simulink model "PortMapTest"  (R2019b)
settings: Solver=FixedStepDiscrete  StartTime=0.0  StopTime=10.0  FixedStep=0.02  RelTol=1e-3
libraries: hdlsllib x4
settings Model: Creator=Yinglongli  LastModifiedBy=Yinglongli
settings OptimizationCC: OptimizeBlockIOStorage=off  BufferReuse=off  GlobalBufferReuse=off  ExpressionFolding=off  LocalBlockOutputs=off  OptimizeDataStoreBuffers=off  BusAssignmentInplaceUpdate=off
settings DebuggingCC: SFUnexpectedBacktrackingDiag=warning  SFNoUnconditionalDefaultTransitionDiag=warning
settings RTWCC: GenerateReport=on  BuildConfiguration=Debug  LaunchReport=on
settings CodeAppCC: ForceParamTrailComments=on  MATLABSourceComments=on  EnableCustomComments=on
settings GRTTargetCC: CombineSignalStateStructs=on  SupportVariableSizeSignals=on  MultiInstanceErrorCode=Warning

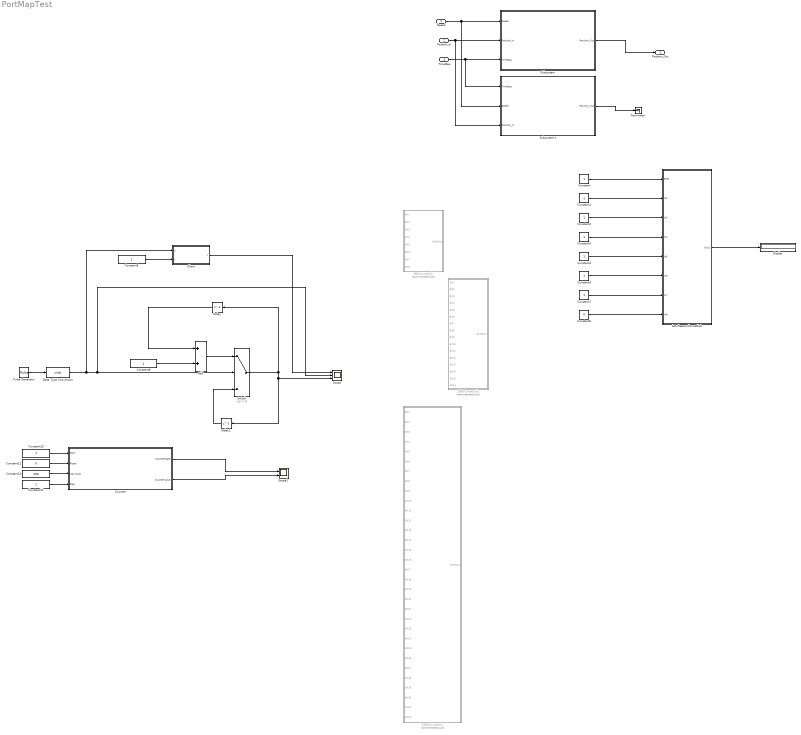
== system PortMapTest ==
  Speed : Inport
  Position_In : Inport  Port=2
  TimeGap : Inport  Port=3
  16BitConcatSub : Subsystem  Commented=on
  32BitConcatSub : Subsystem  Commented=on
  8BitConcatSub : Subsystem  Commented=on
  ActvReasonConcatSub : Subsystem  mask{numInputs=8}
      mask prompts: numInputs "Number of Inputs"
      mask TypeOptions numInputs: Bit Concat/numInputs
      mask Callback numInputs: parentInHandle = find_system(gcb,'FindAll','on','SearchDepth','1','BlockType','Inport');
      mask Display: disp('Bit Concatenation\n')
  Add : Sum
  Chart : Stateflow chart  BlockKeywords=__PRM__SERIALIZED__DATA__:Stateflow Chart,Stateflow Diagram  TreatAsAtomicUnit=on
  Constant{,1..5,7} (7 alike) : Constant  OutDataTypeStr=boolean
  Constant10 : Constant  Value=200  OutDataTypeStr=uint32
  Constant11 : Constant  OutDataTypeStr=uint8
  Constant12 : Constant  Value=0  OutDataTypeStr=uint8
  Constant13 : Constant  OutDataTypeStr=uint8
  Constant6 : Constant  Value=0  OutDataTypeStr=boolean
  Constant8 : Constant
  Constant9 : Constant  OutDataTypeStr=uint32
  Counter : Subsystem
  Data Type Conversion : DataTypeConversion  OutDataTypeStr=uint8
  Delay : Delay  DelayLength=1
  Delay1 : Delay  DelayLength=1
  Display : Display
      settings: Format=decimal (Stored Integer)
  Pulse Generator : DiscretePulseGenerator  PulseType=Time based  Period=0.04  PulseWidth=50
  Scope : Scope  NumInputPorts=3
  Scope1 : Scope  NumInputPorts=2
  Subsystem : Subsystem
  Subsystem1 : Subsystem
  Switch : Switch  Criteria=u2 > Threshold
  Terminator : Terminator
  Position_Out : Outport
  wires:
  Speed/1 -> Subsystem/1(Speed), Subsystem1/2(Speed)
  Position_In/1 -> Subsystem/2(Position_In), Subsystem1/3(Position_In)
  TimeGap/1 -> Subsystem/3(TimeGap), Subsystem1/1(TimeGap)
  Subsystem/1(Position_Out) -> Position_Out/1
  Subsystem1/1(Position_Out) -> Terminator/1
  Constant/1 -> ActvReasonConcatSub/1(Bit8)
  Constant1/1 -> ActvReasonConcatSub/2(In2)
  Constant2/1 -> ActvReasonConcatSub/3(In3)
  Constant3/1 -> ActvReasonConcatSub/4(In4)
  Constant4/1 -> ActvReasonConcatSub/5(In5)
  Constant5/1 -> ActvReasonConcatSub/6(In6)
  Constant7/1 -> ActvReasonConcatSub/7(In7)
  Constant6/1 -> ActvReasonConcatSub/8(In8)
  ActvReasonConcatSub/1(Out1) -> Display/1
  Constant8/1 -> Add/2
  Delay/1 -> Add/1
  Add/1 -> Switch/1
  Switch/1 -> Scope/3, Delay1/1, Delay/1
  Delay1/1 -> Switch/3
  Chart/1(y) -> Scope/1
  Pulse Generator/1 -> Data Type Conversion/1
  Constant9/1 -> Chart/2(t)
  Data Type Conversion/1 -> Chart/1(u), Scope/2, Switch/2
  Constant10/1 -> Counter/3(MaxValue)
  Constant11/1 -> Counter/4(Step)
  Constant12/1 -> Counter/2(Reset)
  Constant13/1 -> Counter/1(Start)
  Counter/1(CounterState) -> Scope1/1
  Counter/2(CounterValue) -> Scope1/2

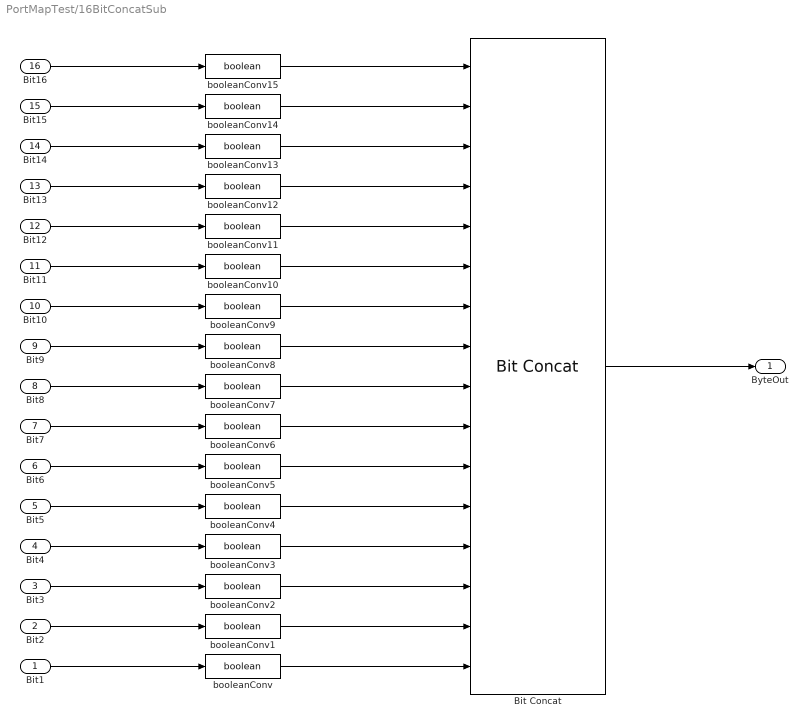
== system PortMapTest/16BitConcatSub ==
  Bit1 : Inport
  Bit2 : Inport  Port=2
  Bit3 : Inport  Port=3
  Bit4 : Inport  Port=4
  Bit5 : Inport  Port=5
  Bit6 : Inport  Port=6
  Bit7 : Inport  Port=7
  Bit8 : Inport  Port=8
  Bit9 : Inport  Port=9
  Bit10 : Inport  Port=10
  Bit11 : Inport  Port=11
  Bit12 : Inport  Port=12
  Bit13 : Inport  Port=13
  Bit14 : Inport  Port=14
  Bit15 : Inport  Port=15
  Bit16 : Inport  Port=16
  Bit Concat : hdlsllib/Logic and Bit Operations/Bit Concat  numInputs=16
      settings: SourceProductName=Simulink
  booleanConv{,1..15} (16 alike) : DataTypeConversion  OutDataTypeStr=boolean
  ByteOut : Outport
  wires:
  Bit Concat/1 -> ByteOut/1
  Bit8/1 -> booleanConv7/1
  Bit7/1 -> booleanConv6/1
  Bit6/1 -> booleanConv5/1
  Bit5/1 -> booleanConv4/1
  Bit4/1 -> booleanConv3/1
  Bit3/1 -> booleanConv2/1
  Bit2/1 -> booleanConv1/1
  Bit1/1 -> booleanConv/1
  booleanConv7/1 -> Bit Concat/9
  booleanConv6/1 -> Bit Concat/10
  booleanConv5/1 -> Bit Concat/11
  booleanConv4/1 -> Bit Concat/12
  booleanConv3/1 -> Bit Concat/13
  booleanConv2/1 -> Bit Concat/14
  booleanConv1/1 -> Bit Concat/15
  booleanConv/1 -> Bit Concat/16
  booleanConv15/1 -> Bit Concat/1
  booleanConv14/1 -> Bit Concat/2
  booleanConv13/1 -> Bit Concat/3
  booleanConv12/1 -> Bit Concat/4
  booleanConv11/1 -> Bit Concat/5
  booleanConv10/1 -> Bit Concat/6
  booleanConv9/1 -> Bit Concat/7
  booleanConv8/1 -> Bit Concat/8
  Bit16/1 -> booleanConv15/1
  Bit15/1 -> booleanConv14/1
  Bit14/1 -> booleanConv13/1
  Bit13/1 -> booleanConv12/1
  Bit12/1 -> booleanConv11/1
  Bit10/1 -> booleanConv9/1
  Bit11/1 -> booleanConv10/1
  Bit9/1 -> booleanConv8/1

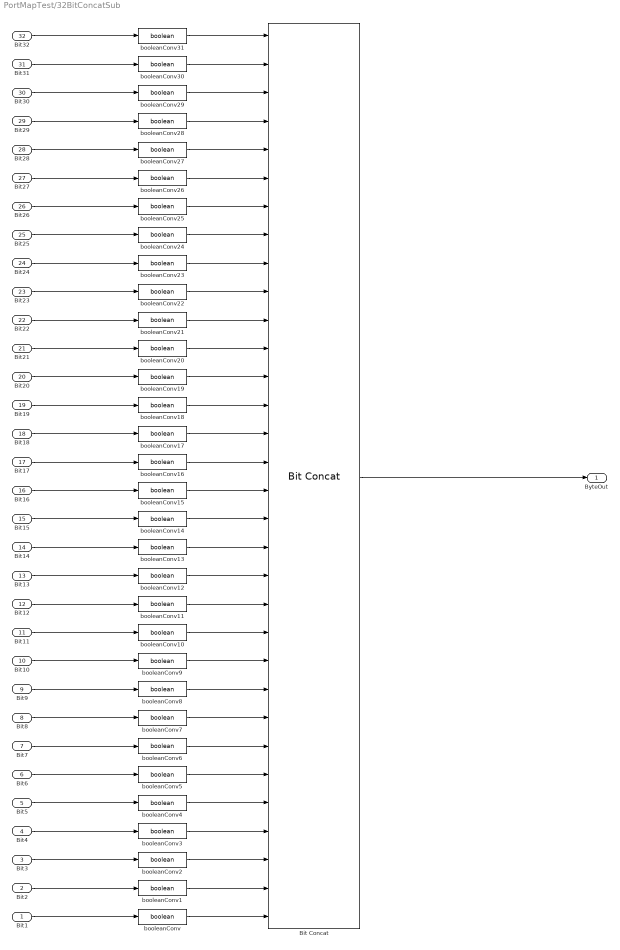
== system PortMapTest/32BitConcatSub ==
  Bit1 : Inport
  Bit2 : Inport  Port=2
  Bit3 : Inport  Port=3
  Bit4 : Inport  Port=4
  Bit5 : Inport  Port=5
  Bit6 : Inport  Port=6
  Bit7 : Inport  Port=7
  Bit8 : Inport  Port=8
  Bit9 : Inport  Port=9
  Bit10 : Inport  Port=10
  Bit11 : Inport  Port=11
  Bit12 : Inport  Port=12
  Bit13 : Inport  Port=13
  Bit14 : Inport  Port=14
  Bit15 : Inport  Port=15
  Bit16 : Inport  Port=16
  Bit17 : Inport  Port=17
  Bit18 : Inport  Port=18
  Bit19 : Inport  Port=19
  Bit20 : Inport  Port=20
  Bit21 : Inport  Port=21
  Bit22 : Inport  Port=22
  Bit23 : Inport  Port=23
  Bit24 : Inport  Port=24
  Bit25 : Inport  Port=25
  Bit26 : Inport  Port=26
  Bit27 : Inport  Port=27
  Bit28 : Inport  Port=28
  Bit29 : Inport  Port=29
  Bit30 : Inport  Port=30
  Bit31 : Inport  Port=31
  Bit32 : Inport  Port=32
  Bit Concat : hdlsllib/Logic and Bit Operations/Bit Concat  numInputs=32
      settings: SourceProductName=Simulink
  booleanConv{,1..31} (32 alike) : DataTypeConversion  OutDataTypeStr=boolean
  ByteOut : Outport
  wires:
  Bit Concat/1 -> ByteOut/1
  Bit8/1 -> booleanConv7/1
  Bit7/1 -> booleanConv6/1
  Bit6/1 -> booleanConv5/1
  Bit5/1 -> booleanConv4/1
  Bit4/1 -> booleanConv3/1
  Bit3/1 -> booleanConv2/1
  Bit2/1 -> booleanConv1/1
  Bit1/1 -> booleanConv/1
  Bit16/1 -> booleanConv15/1
  Bit15/1 -> booleanConv14/1
  Bit14/1 -> booleanConv13/1
  Bit13/1 -> booleanConv12/1
  Bit12/1 -> booleanConv11/1
  Bit10/1 -> booleanConv9/1
  Bit11/1 -> booleanConv10/1
  Bit9/1 -> booleanConv8/1
  booleanConv/1 -> Bit Concat/32
  booleanConv1/1 -> Bit Concat/31
  booleanConv2/1 -> Bit Concat/30
  booleanConv3/1 -> Bit Concat/29
  booleanConv4/1 -> Bit Concat/28
  booleanConv5/1 -> Bit Concat/27
  booleanConv6/1 -> Bit Concat/26
  booleanConv7/1 -> Bit Concat/25
  booleanConv8/1 -> Bit Concat/24
  booleanConv9/1 -> Bit Concat/23
  booleanConv10/1 -> Bit Concat/22
  booleanConv11/1 -> Bit Concat/21
  booleanConv12/1 -> Bit Concat/20
  booleanConv13/1 -> Bit Concat/19
  booleanConv14/1 -> Bit Concat/18
  booleanConv15/1 -> Bit Concat/17
  booleanConv31/1 -> Bit Concat/1
  booleanConv30/1 -> Bit Concat/2
  booleanConv29/1 -> Bit Concat/3
  booleanConv28/1 -> Bit Concat/4
  booleanConv27/1 -> Bit Concat/5
  booleanConv26/1 -> Bit Concat/6
  booleanConv25/1 -> Bit Concat/7
  booleanConv24/1 -> Bit Concat/8
  booleanConv23/1 -> Bit Concat/9
  booleanConv22/1 -> Bit Concat/10
  booleanConv21/1 -> Bit Concat/11
  booleanConv20/1 -> Bit Concat/12
  booleanConv19/1 -> Bit Concat/13
  booleanConv18/1 -> Bit Concat/14
  booleanConv17/1 -> Bit Concat/15
  booleanConv16/1 -> Bit Concat/16
  Bit17/1 -> booleanConv16/1
  Bit18/1 -> booleanConv17/1
  Bit19/1 -> booleanConv18/1
  Bit20/1 -> booleanConv19/1
  Bit21/1 -> booleanConv20/1
  Bit22/1 -> booleanConv21/1
  Bit23/1 -> booleanConv22/1
  Bit24/1 -> booleanConv23/1
  Bit25/1 -> booleanConv24/1
  Bit26/1 -> booleanConv25/1
  Bit27/1 -> booleanConv26/1
  Bit28/1 -> booleanConv27/1
  Bit29/1 -> booleanConv28/1
  Bit30/1 -> booleanConv29/1
  Bit31/1 -> booleanConv30/1
  Bit32/1 -> booleanConv31/1

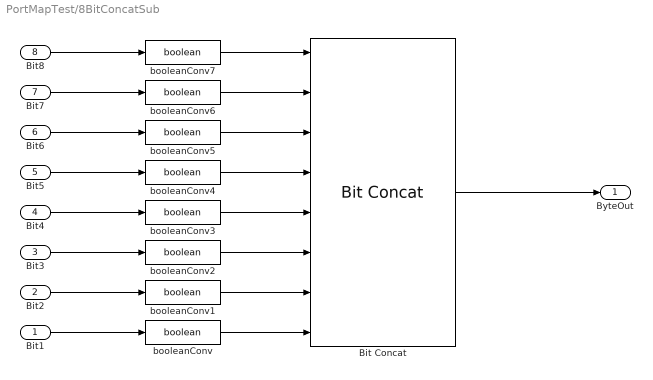
== system PortMapTest/8BitConcatSub ==
  Bit1 : Inport
  Bit2 : Inport  Port=2
  Bit3 : Inport  Port=3
  Bit4 : Inport  Port=4
  Bit5 : Inport  Port=5
  Bit6 : Inport  Port=6
  Bit7 : Inport  Port=7
  Bit8 : Inport  Port=8
  Bit Concat : hdlsllib/Logic and Bit Operations/Bit Concat  numInputs=8
      settings: SourceProductName=Simulink
  booleanConv{,1..7} (8 alike) : DataTypeConversion  OutDataTypeStr=boolean
  ByteOut : Outport
  wires:
  Bit Concat/1 -> ByteOut/1
  Bit8/1 -> booleanConv7/1
  Bit7/1 -> booleanConv6/1
  Bit6/1 -> booleanConv5/1
  Bit5/1 -> booleanConv4/1
  Bit4/1 -> booleanConv3/1
  Bit3/1 -> booleanConv2/1
  Bit2/1 -> booleanConv1/1
  Bit1/1 -> booleanConv/1
  booleanConv/1 -> Bit Concat/8
  booleanConv1/1 -> Bit Concat/7
  booleanConv2/1 -> Bit Concat/6
  booleanConv3/1 -> Bit Concat/5
  booleanConv4/1 -> Bit Concat/4
  booleanConv5/1 -> Bit Concat/3
  booleanConv6/1 -> Bit Concat/2
  booleanConv7/1 -> Bit Concat/1

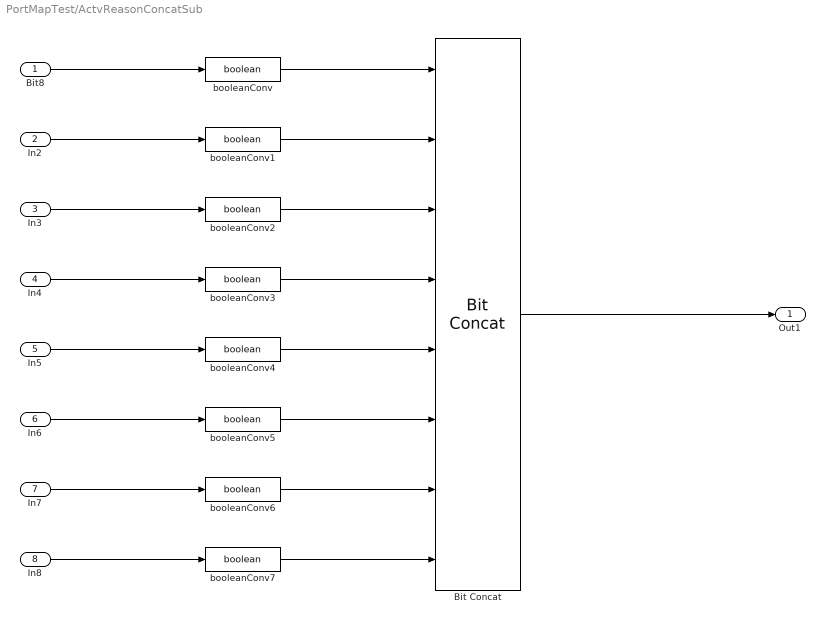
== system PortMapTest/ActvReasonConcatSub ==
  Bit8 : Inport
  In2 : Inport  Port=2
  In3 : Inport  Port=3
  In4 : Inport  Port=4
  In5 : Inport  Port=5
  In6 : Inport  Port=6
  In7 : Inport  Port=7
  In8 : Inport  Port=8
  Bit Concat : hdlsllib/Logic and Bit Operations/Bit Concat  numInputs=numInputs
      settings: SourceProductName=Simulink
  booleanConv{,1..7} (8 alike) : DataTypeConversion  OutDataTypeStr=boolean
  Out1 : Outport
  wires:
  In8/1 -> booleanConv7/1
  In2/1 -> booleanConv1/1
  In6/1 -> booleanConv5/1
  Bit Concat/1 -> Out1/1
  Bit8/1 -> booleanConv/1
  In7/1 -> booleanConv6/1
  In5/1 -> booleanConv4/1
  In4/1 -> booleanConv3/1
  In3/1 -> booleanConv2/1
  booleanConv/1 -> Bit Concat/1
  booleanConv1/1 -> Bit Concat/2
  booleanConv2/1 -> Bit Concat/3
  booleanConv3/1 -> Bit Concat/4
  booleanConv4/1 -> Bit Concat/5
  booleanConv5/1 -> Bit Concat/6
  booleanConv6/1 -> Bit Concat/7
  booleanConv7/1 -> Bit Concat/8

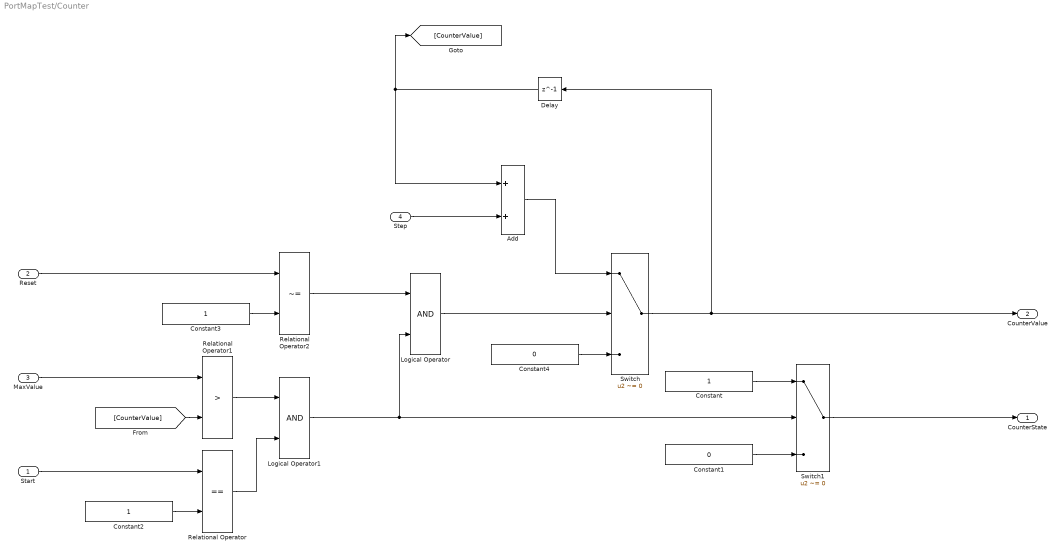
== system PortMapTest/Counter ==
  Start : Inport  OutDataTypeStr=uint8
  Reset : Inport  Port=2  OutDataTypeStr=uint8
  MaxValue : Inport  Port=3  OutDataTypeStr=uint32
  Step : Inport  Port=4  OutDataTypeStr=uint8
  Add : Sum
  Constant : Constant  OutDataTypeStr=uint8
  Constant1 : Constant  Value=0  OutDataTypeStr=uint8
  Constant2 : Constant  OutDataTypeStr=uint8
  Constant3 : Constant  OutDataTypeStr=uint8
  Constant4 : Constant  Value=0  OutDataTypeStr=uint32
  Delay : Delay  DelayLength=1
  Logical Operator : Logic  AllPortsSameDT=off  OutDataTypeStr=boolean
  Logical Operator1 : Logic  AllPortsSameDT=off  OutDataTypeStr=boolean
  Relational Operator : RelationalOperator  Operator===  OutDataTypeStr=boolean  RndMeth=Simplest
  Relational Operator1 : RelationalOperator  Operator=>  OutDataTypeStr=boolean  RndMeth=Simplest
  Relational Operator2 : RelationalOperator  Operator=~=  OutDataTypeStr=boolean  RndMeth=Simplest
  Switch : Switch  Criteria=u2 ~= 0  OutDataTypeStr=uint32
  Switch1 : Switch  Criteria=u2 ~= 0
  CounterState : Outport  OutDataTypeStr=uint8
  CounterValue : Outport  Port=2  OutDataTypeStr=uint32
  wires:
  Add/1 -> Switch/1
  Delay/1 -> [CounterValue], Add/1
  Start/1 -> Relational Operator/1
  Logical Operator1/1 -> Switch1/2, Logical Operator/2
  Switch1/1 -> CounterState/1
  Constant/1 -> Switch1/1
  Constant1/1 -> Switch1/3
  Constant2/1 -> Relational Operator/2
  Constant3/1 -> Relational Operator2/2
  Reset/1 -> Relational Operator2/1
  Logical Operator/1 -> Switch/2
  Switch/1 -> CounterValue/1, Delay/1
  MaxValue/1 -> Relational Operator1/1
  [CounterValue] -> Relational Operator1/2
  Constant4/1 -> Switch/3
  Relational Operator1/1 -> Logical Operator1/1
  Relational Operator/1 -> Logical Operator1/2
  Relational Operator2/1 -> Logical Operator/1
  Step/1 -> Add/2

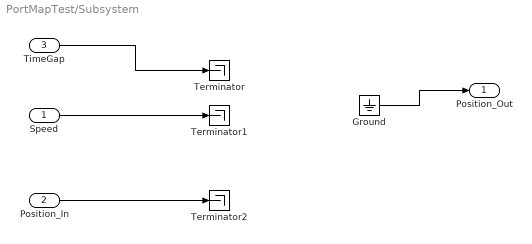
== system PortMapTest/Subsystem ==
  Speed : Inport
  Position_In : Inport  Port=2
  TimeGap : Inport  Port=3
  Ground : Ground
  Terminator : Terminator
  Terminator1 : Terminator
  Terminator2 : Terminator
  Position_Out : Outport
  wires:
  TimeGap/1 -> Terminator/1
  Speed/1 -> Terminator1/1
  Position_In/1 -> Terminator2/1
  Ground/1 -> Position_Out/1

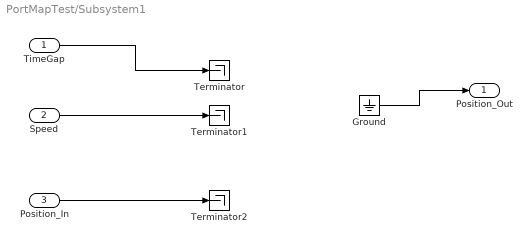
== system PortMapTest/Subsystem1 ==
  TimeGap : Inport
  Speed : Inport  Port=2
  Position_In : Inport  Port=3
  Ground : Ground
  Terminator : Terminator
  Terminator1 : Terminator
  Terminator2 : Terminator
  Position_Out : Outport
  wires:
  Ground/1 -> Position_Out/1
  Position_In/1 -> Terminator2/1
  Speed/1 -> Terminator1/1
  TimeGap/1 -> Terminator/1

== stateflow chart PortMapTest/Chart ==
  state On
    en: y = y + t;
    du: y = y + t;
  state Off
    en: y = y;
  (default) -> (junction 1)
  (junction 1) -> Off [order 2]
  (junction 1) -> On [order 1] : [u>0]
  On -> Off : [u<=0]
  Off -> On : [u>0]
  data: u input uint8; y output uint32 =uint32(0); t input uint32
